simulink model "mode_lame_2019b"  (R2020a)
settings: Solver=VariableStepAuto  StartTime=0.0  StopTime=10  RelTol=1e-3
libraries: simulink x1
settings Model: Creator=antoi  LastModifiedBy=antoi
settings DebuggingCC: UnderSpecifiedDimensionMsg=warning

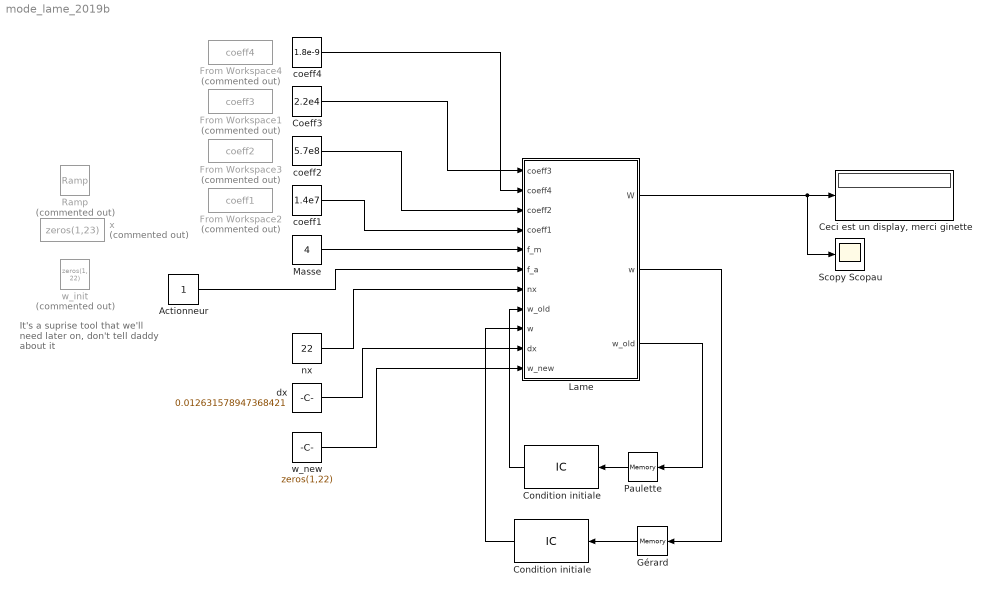
== system mode_lame_2019b ==
  note: It's a suprise tool that we'll need later on, don't tell daddy about it
  Actionneur : Constant
  "Ceci est un display, merci ginette" : Display
  Coeff3 : Constant  Value=2.2e4
  Condition initiale : InitialCondition  Value=zeros(1,22)
  "Condition initiale " : InitialCondition  Value=zeros(1,22)
  From Workspace1 : FromWorkspace  Commented=on  VariableName=coeff3
  From Workspace2 : FromWorkspace  Commented=on  VariableName=coeff1
  From Workspace3 : FromWorkspace  Commented=on  VariableName=coeff2
  From Workspace4 : FromWorkspace  Commented=on  VariableName=coeff4
  Gérard : Memory
  Lame : MATLAB Function  TreatAsAtomicUnit=on
  Masse : Constant  Value=4
  Paulette : Memory
  Ramp : simulink/Sources/Ramp  Commented=on  slope=1  start=0  InitialOutput=0
  Scopy Scopau : Scope
  coeff1 : Constant  Value=1.4e7
  coeff2 : Constant  Value=5.7e8
  coeff4 : Constant  Value=1.8e-9
  dx : Constant  Value=0.012631578947368421
  nx : Constant  Value=22
  w_init : Constant  Commented=on  Value=zeros(1, 22)
  w_new : Constant  Value=zeros(1,22)
  x : FromWorkspace  Commented=on  VariableName=zeros(1,23)
  wires:
  Masse/1 -> Lame/5(f_m)
  Lame/2(w) -> Gérard/1
  Lame/3(w_old) -> Paulette/1
  Gérard/1 -> Condition initiale/1
  Paulette/1 -> "Condition initiale "/1
  Lame/1(W) -> Scopy Scopau/1, "Ceci est un display, merci ginette"/1
  Coeff3/1 -> Lame/1(coeff3)
  coeff4/1 -> Lame/2(coeff4)
  nx/1 -> Lame/7(nx)
  "Condition initiale "/1 -> Lame/8("w_old ")
  Condition initiale/1 -> Lame/9("w ")
  coeff2/1 -> Lame/3(coeff2)
  dx/1 -> Lame/10(dx)
  w_new/1 -> Lame/11(w_new)
  Actionneur/1 -> Lame/6(f_a)
  coeff1/1 -> Lame/4(coeff1)

== matlab function mode_lame_2019b/Lame ==
  data: coeff3 input; coeff4 input; coeff2 input; coeff1 input; f_m input; W output; f_a input; nx input; w_old input; w input; dx input; w output; w_old output; w_new input
function [W, w, w_old] = fcn(coeff3, coeff4, coeff2, coeff1, f_m, f_a, nx, w_old, w, dx, w_new) 
    
    % Vecteur position
    %w_new = zeros(1,nx); %PO y dit non non non
    
    
    % La force
    F = zeros(1, nx);
    F(11) = f_a + f_m;
    
    
%     h = plot(x, w_init, x, w_new);
%     xlabel("X [m]")
%     ylabel("Déflexion [m]")
%     ylim([-0.01,0.01])
%     grid on

    
    for i = 3:nx-2
        
        %Équation différentielle résolue par Sam
        w_new(i) = (-coeff1*(w(i+2)-4*w(i+1)+6*w(i)-4*w(i-1)+w(i-2)) - coeff2*(-2*w(i)+w_old(i)) + coeff3*w(i) + F(i)/dx)*coeff4;

        %% Conditions limites 
        w_new(1:2) =0;                 % Clampé à zero, position et dérivée nulle (le bout de la lame est fixe)

        w_new(end-1) = 2*w_new(end-2)-w_new(end-3);    % Libre au bout dérivées 2e et 3e nulles
        w_new(end) = 2*w_new(end-1)-w_new(end-2);
        
%         set(h(2), "Ydata", w_new);
%         drawnow
    end
     
    %% Préparation du prochain tour
    
    w_old = w;
    w = w_new;
    W = w(end);
end
